simulink model "prblm3"  (R2020b)
settings: Solver=VariableStepAuto  StartTime=0.0  StopTime=10.0  RelTol=1e-3
undefined symbols (not defined in the file): b, m
settings Model: Creator=Shree  LastModifiedBy=Shree

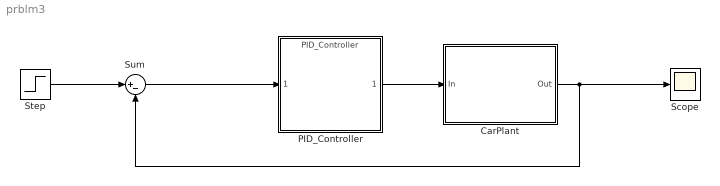
== system prblm3 ==
  CarPlant : Subsystem
  PID_Controller : ModelReference  ModelNameDialog=PID_Controller  UsingDefaultArgumentValue=0,0,0  SimulationMode=Normal  ModelReferenceVersion=1.10
  Scope : Scope
  Step : Step  After=10  SampleTime=0
  Sum : Sum  Inputs=|+-
  wires:
  CarPlant/1(Out) -> Scope/1, Sum/2
  Step/1 -> Sum/1
  PID_Controller/1 -> CarPlant/1(In)
  Sum/1 -> PID_Controller/1

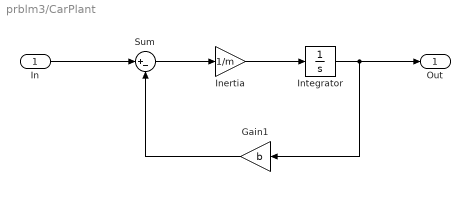
== system prblm3/CarPlant ==
  In : Inport
  Gain1 : Gain  Gain=b
  Inertia : Gain  Gain=1/m
  Integrator : Integrator
  Sum : Sum  Inputs=|+-
  Out : Outport
  wires:
  Inertia/1 -> Integrator/1
  Integrator/1 -> Out/1, Gain1/1
  Sum/1 -> Inertia/1
  Gain1/1 -> Sum/2
  In/1 -> Sum/1
